simulink model "mg_simulator"  (Simulink 9.0)
settings: Solver=VariableStepAuto  StartTime=0.0  StopTime=Tsim  FixedStep=.005  MaxStep=Ts  RelTol=1e-6  EnableMultiTasking=on
InitFcn:
  | mg_simulator_init
values from neighbouring files (symbols this model uses):
  g_vector = zeros(1,4)    [mg_simulator_init.m]
  Init = [100; 200; 300; 400]    [mg_simulator_init.m]
  N = 2    [mg_simulator_init.m]
  n_Qi = total(2)    [estimator_pflow_dynamics.m]    (also in estimator_pflow_dynamics2.m; mg_simulator_init.m = 4.24e-4*ones(1,4))
  Q = 5*eye    [mg_simulator_init.m]
  Q_di = total(4)    [estimator_pflow_dynamics.m]    (also in estimator_pflow_dynamics2.m; mg_simulator_init.m = 0*ones(1,4))
  Q_Li = 0*ones(1,4)    [mg_simulator_init.m]
  R = 1*eye    [mg_simulator_init.m]
  Thresh = 1    [mg_simulator_init.m]
  Ts = total(7)    [estimator_pflow_dynamics.m]    (also in estimator_pflow_dynamics2.m = total(8); mg_simulator_init.m = 0.005)
  v_ref = 310    [mg_simulator_init.m]
  W = 10*eye    [mg_simulator_init.m]
  w_noise_est = w_noise    [mg_simulator_init.m]
undefined symbols (not defined in the file or in its folder): mpc_run_nodewise_mdl_fast, mpc_run_nodewise_mdl_fast2, mpc_run_nodewise_mdl_fast3, plecs
libraries: sharedTrackingLibrary x4
settings Model: SuppressorTable=22 serialization::archive 11 0 6 0 0 0 0 0  Creator=manaswini  LastModifiedBy=seananderson  ExtModeAutoUpdateStatusClock=off
settings DataIOCC: LimitDataPoints=on  SignalLoggingSaveFormat=ModelDataLogs
settings OptimizationCC: ExpressionDepthLimit=2147483647
settings DebuggingCC: AlgebraicLoopMsg=none  SaveWithParameterizedLinksMsg=none  MaxConsecutiveZCsMsg=none  SolverPrmCheckMsg=warning  FcnCallInpInsideContextMsg=warning  StateNameClashWarn=warning
settings HardwareCC: TargetHWDeviceType=32-bit Generic
settings GRTTargetCC: TargetFcnLib=ansi_tfl_tmw.mat  CombineOutputUpdateFcns=off  GRTInterface=on

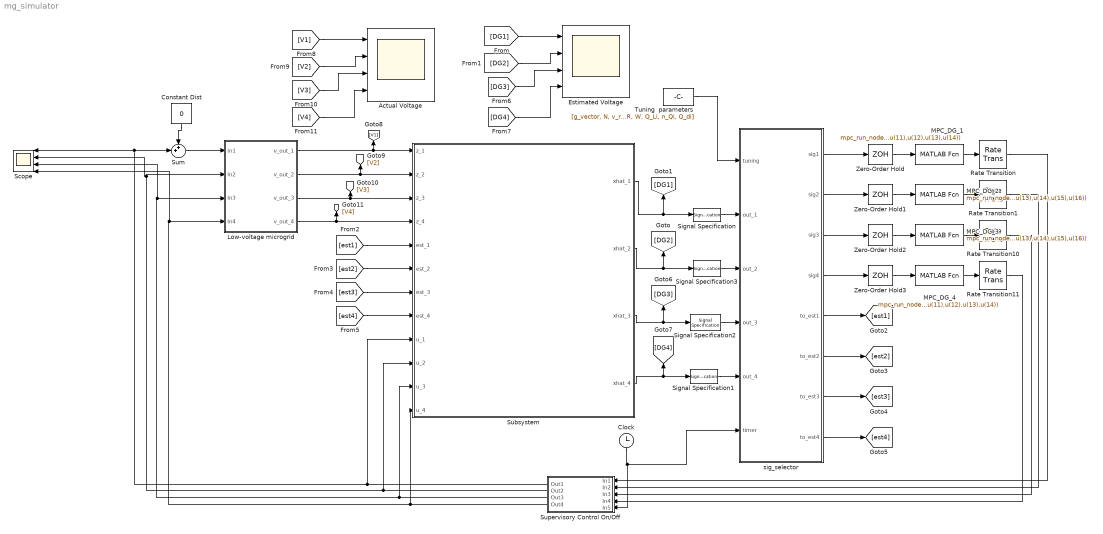
== system mg_simulator ==
  Actual Voltage : Scope  NumInputPorts=4
  Clock : Clock
  Constant Dist : Constant  Value=0
  Estimated Voltage : Scope  NumInputPorts=4
  Low-voltage microgrid : Subsystem  LoadFcn=plecs('sl', 200);  InitFcn=plecs('sl', 214);  StartFcn=plecs('sl', 208);  StopFcn=plecs('sl', 209);  mask(PlecsCircuit){PLECSData=<binary blob, 37876 chars, not shown>}
      mask prompts: PLECSData "PLECS Data (Do not delete or modify!)"
      mask init:
      | % PLACE CUSTOM INITIALIZATIONS ABOVE
      | % DO NOT REMOVE
      | plecs('sl', 215);
      | % DO NOT REMOVE
      settings: CopyFcn=plecs('sl', 203);  DeleteFcn=plecs('sl', 205);  UndoDeleteFcn=plecs('sl', 206);  PreSaveFcn=plecs('sl', 211);  PostSaveFcn=plecs('sl', 201);  NameChangeFcn=plecs('sl', 210);  DestroyFcn=plecs('sl', 207);  PreCopyFcn=plecs('sl', 216);  OpenFcn=plecs('sl', 202);  ErrorFcn=plerrorfcn
      mask Help: web(['file:///' fullfile(plecsdoc, 'creatingacircuit.html')])
      mask Display: disp('PLECS\nCircuit')
  MPC_DG_1 : MATLABFcn  MATLABFcn=mpc_run_nodewise_mdl_fast(u(1),u(2),u(3),u(4),u(5),u(6),u(7),u(8),u(9),u(10),u(11),u(12),u(13),u(14))  SampleTime=Ts
  MPC_DG_2 : MATLABFcn  MATLABFcn=mpc_run_nodewise_mdl_fast2(u(1),u(2:3),u(4:5),u(6),u(7),u(8),u(9),u(10),u(11),u(12),u(13),u(14),u(15),u(16))  SampleTime=Ts
  MPC_DG_3 : MATLABFcn  MATLABFcn=mpc_run_nodewise_mdl_fast3(u(1),u(2:3),u(4:5),u(6),u(7),u(8),u(9),u(10),u(11),u(12),u(13),u(14),u(15),u(16))  SampleTime=Ts
  MPC_DG_4 : MATLABFcn  MATLABFcn=mpc_run_nodewise_mdl_fast(u(1),u(2),u(3),u(4),u(5),u(6),u(7),u(8),u(9),u(10),u(11),u(12),u(13),u(14))  SampleTime=Ts
  Rate Transition{,1,10..11} (4 alike) : RateTransition  OutPortSampleTimeOpt=Inherit  OutPortSampleTime=Ts
  Scope : Scope  NumInputPorts=4
  Signal Specification : SignalSpecification  Dimensions=[ 1 2]
  Signal Specification1 : SignalSpecification  Dimensions=[ 1 2]
  Signal Specification2 : SignalSpecification  Dimensions=[ 1 3]
  Signal Specification3 : SignalSpecification  Dimensions=[ 1 3]
  Subsystem : Subsystem
  Sum : Sum  Inputs=++|
  Supervisory Control On/Off : Subsystem
  Tuning  parameters : Constant  Value=[g_vector, N, v_ref, Ts, Q, R, W, Q_Li, n_Qi, Q_di]
  Zero-Order Hold{,1..3} (4 alike) : ZeroOrderHold  SampleTime=Ts
  sig_selector : MATLAB Function  TreatAsAtomicUnit=on
  wires:
  Clock/1 -> sig_selector/6(timer), Supervisory Control On/Off/5(In5)
  Tuning  parameters/1 -> sig_selector/1(tuning)
  Zero-Order Hold/1 -> MPC_DG_1/1
  sig_selector/1(sig1) -> Zero-Order Hold/1
  MPC_DG_1/1 -> Rate Transition/1
  Rate Transition/1 -> Supervisory Control On/Off/1(In1)
  MPC_DG_2/1 -> Rate Transition1/1
  sig_selector/2(sig2) -> Zero-Order Hold1/1
  Rate Transition1/1 -> Supervisory Control On/Off/2(In2)
  [DG1] -> Estimated Voltage/1
  [DG2] -> Estimated Voltage/2
  sig_selector/5(to_est1) -> [est1]
  sig_selector/6(to_est2) -> [est2]
  Zero-Order Hold1/1 -> MPC_DG_2/1
  Supervisory Control On/Off/1(Out1) -> Subsystem/9(u_1), Sum/2, Scope/1
  Supervisory Control On/Off/2(Out2) -> Subsystem/10(u_2), Low-voltage microgrid/2(In2), Scope/2
  Zero-Order Hold2/1 -> MPC_DG_3/1
  sig_selector/3(sig3) -> Zero-Order Hold2/1
  MPC_DG_3/1 -> Rate Transition10/1
  Zero-Order Hold3/1 -> MPC_DG_4/1
  sig_selector/4(sig4) -> Zero-Order Hold3/1
  MPC_DG_4/1 -> Rate Transition11/1
  sig_selector/7(to_est3) -> [est3]
  sig_selector/8(to_est4) -> [est4]
  Rate Transition10/1 -> Supervisory Control On/Off/3(In3)
  Rate Transition11/1 -> Supervisory Control On/Off/4(In4)
  Supervisory Control On/Off/3(Out3) -> Subsystem/11(u_3), Low-voltage microgrid/3(In3), Scope/3
  Supervisory Control On/Off/4(Out4) -> Subsystem/12(u_4), Low-voltage microgrid/4(In4), Scope/4
  Subsystem/2(xhat_2) -> Signal Specification3/1, [DG2]
  Low-voltage microgrid/1(v_out_1) -> [V1], Subsystem/1(z_1)
  Low-voltage microgrid/3(v_out_3) -> [V3], Subsystem/3(z_3)
  Low-voltage microgrid/4(v_out_4) -> [V4], Subsystem/4(z_4)
  [est1] -> Subsystem/5(est_1)
  [est2] -> Subsystem/6(est_2)
  [est3] -> Subsystem/7(est_3)
  [est4] -> Subsystem/8(est_4)
  Subsystem/4(xhat_4) -> Signal Specification1/1, [DG4]
  Subsystem/3(xhat_3) -> Signal Specification2/1, [DG3]
  [DG3] -> Estimated Voltage/3
  [DG4] -> Estimated Voltage/4
  Signal Specification/1 -> sig_selector/2(out_1)
  Subsystem/1(xhat_1) -> Signal Specification/1, [DG1]
  Signal Specification1/1 -> sig_selector/5(out_4)
  Signal Specification2/1 -> sig_selector/4(out_3)
  Signal Specification3/1 -> sig_selector/3(out_2)
  [V4] -> Actual Voltage/4
  [V3] -> Actual Voltage/3
  [V1] -> Actual Voltage/1
  [V2] -> Actual Voltage/2
  Low-voltage microgrid/2(v_out_2) -> [V2], Subsystem/2(z_2)
  Sum/1 -> Low-voltage microgrid/1(In1)
  Constant Dist/1 -> Sum/1

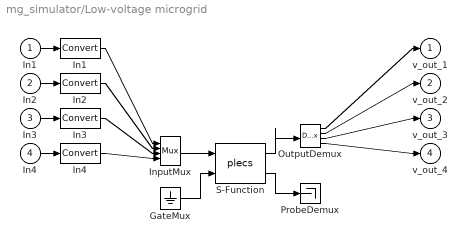
== system mg_simulator/Low-voltage microgrid ==
  In1 : Inport  PortDimensions=1
  In2 : Inport  Port=2  PortDimensions=1
  In3 : Inport  Port=3  PortDimensions=1
  In4 : Inport  Port=4  PortDimensions=1
  " GateMux " : Ground
  " In1 " : DataTypeConversion  SaturateOnIntegerOverflow=on  RndMeth=Zero
  " In2 " : DataTypeConversion  SaturateOnIntegerOverflow=on  RndMeth=Zero
  " In3 " : DataTypeConversion  SaturateOnIntegerOverflow=on  RndMeth=Zero
  " In4 " : DataTypeConversion  SaturateOnIntegerOverflow=on  RndMeth=Zero
  " InputMux " : Mux  Inputs=[ 1 1 1 1 ]
  " OutputDemux " : Demux  Outputs=[ 1 1 1 1 ]
  " ProbeDemux " : Terminator
  " S-Function " : S-Function  FunctionName=plecs  SFunctionDeploymentMode=off  EnableBusSupport=off
  v_out_1 : Outport  PortDimensions=1
  v_out_2 : Outport  Port=2  PortDimensions=1
  v_out_3 : Outport  Port=3  PortDimensions=1
  v_out_4 : Outport  Port=4  PortDimensions=1
  wires:
  " S-Function "/2 -> " ProbeDemux "/1
  " GateMux "/1 -> " S-Function "/2
  " InputMux "/1 -> " S-Function "/1
  " S-Function "/1 -> " OutputDemux "/1
  In1/1 -> " In1 "/1
  " In1 "/1 -> " InputMux "/1
  In2/1 -> " In2 "/1
  " In2 "/1 -> " InputMux "/2
  In3/1 -> " In3 "/1
  " In3 "/1 -> " InputMux "/3
  In4/1 -> " In4 "/1
  " In4 "/1 -> " InputMux "/4
  " OutputDemux "/1 -> v_out_1/1
  " OutputDemux "/2 -> v_out_2/1
  " OutputDemux "/3 -> v_out_3/1
  " OutputDemux "/4 -> v_out_4/1

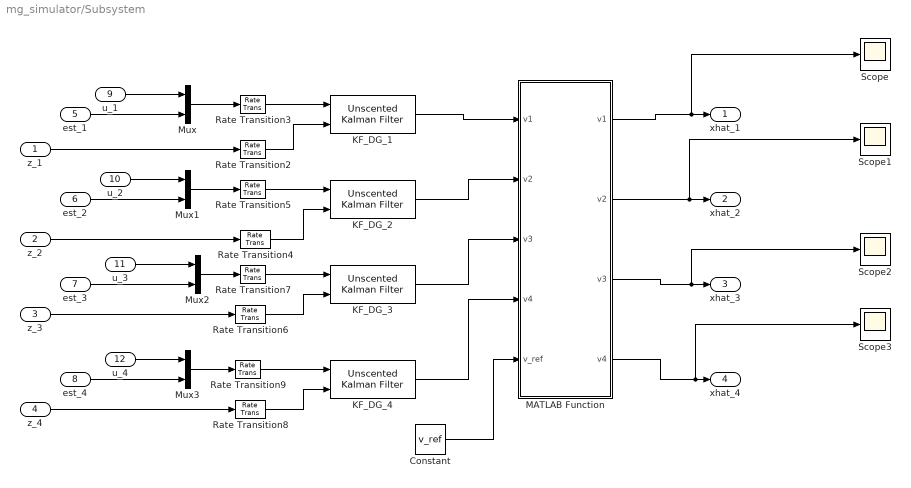
== system mg_simulator/Subsystem ==
  z_1 : Inport
  z_2 : Inport  Port=2
  z_3 : Inport  Port=3
  z_4 : Inport  Port=4
  est_1 : Inport  Port=5
  est_2 : Inport  Port=6
  est_3 : Inport  Port=7
  est_4 : Inport  Port=8
  u_1 : Inport  Port=9
  u_2 : Inport  Port=10
  u_3 : Inport  Port=11
  u_4 : Inport  Port=12
  Constant : Constant  Value=v_ref
  KF_DG_1 : sharedTrackingLibrary/Unscented Kalman Filter  StateTransitionFcn=estimator_pflow_dynamics  HasAdditiveProcessNoise=Nonadditive  ProcessNoise=p_noise_est{i}  HasTimeVaryingProcessNoise=off  HasStateTransitionFcnExtraArgument=1  InitialState=init_state{i}  InitialStateCovariance=p_noise_est{i}  Alpha=1e-1  Beta=2  Kappa=0  MeasurementFcn1=estimator_measurementFcn  HasMeasurementEnablePort1=off  HasAdditiveMeasurementNoise1=Nonadditive  MeasurementNoise1=w_noise_est(i)  HasTimeVaryingMeasurementNoise1=off  HasMeasurementFcnExtraArgument1=0  MeasurementFcn2=myMeasurementFcn  HasMeasurementEnablePort2=off  HasAdditiveMeasurementNoise2=Additive  MeasurementNoise2=1  HasTimeVaryingMeasurementNoise2=off  HasMeasurementFcnExtraArgument2=0  MeasurementFcn3=myMeasurementFcn  HasMeasurementEnablePort3=off  HasAdditiveMeasurementNoise3=Additive  MeasurementNoise3=1  HasTimeVaryingMeasurementNoise3=off  HasMeasurementFcnExtraArgument3=0  MeasurementFcn4=myMeasurementFcn  HasMeasurementEnablePort4=off  HasAdditiveMeasurementNoise4=Additive  MeasurementNoise4=1  HasTimeVaryingMeasurementNoise4=off  HasMeasurementFcnExtraArgument4=0  MeasurementFcn5=myMeasurementFcn  HasMeasurementEnablePort5=off  HasAdditiveMeasurementNoise5=Additive  MeasurementNoise5=1  HasTimeVaryingMeasurementNoise5=off  HasMeasurementFcnExtraArgument5=0  EnableMultirate=off  StateTransitionFcnSampleTime=1  MeasurementFcn1SampleTime=1  MeasurementFcn2SampleTime=1  MeasurementFcn3SampleTime=1  MeasurementFcn4SampleTime=1  MeasurementFcn5SampleTime=1  UseCurrentEstimator=on  OutputStateCovariance=off  DataType=double  SampleTime=Ts  NumberOfMeasurements=1  mask(Unscented Kalman Filter){i=1}
      settings: SourceProductName=Control System Toolbox  SourceProductBaseCode=CT
  KF_DG_2 : sharedTrackingLibrary/Unscented Kalman Filter  StateTransitionFcn=estimator_pflow_dynamics2  HasAdditiveProcessNoise=Nonadditive  ProcessNoise=p_noise_est{i}  HasTimeVaryingProcessNoise=off  HasStateTransitionFcnExtraArgument=1  InitialState=init_state{i}  InitialStateCovariance=p_noise_est{i}  Alpha=1e-1  Beta=2  Kappa=0  MeasurementFcn1=estimator_measurementFcn  HasMeasurementEnablePort1=off  HasAdditiveMeasurementNoise1=Nonadditive  MeasurementNoise1=w_noise_est(i)  HasTimeVaryingMeasurementNoise1=off  HasMeasurementFcnExtraArgument1=0  MeasurementFcn2=myMeasurementFcn  HasMeasurementEnablePort2=off  HasAdditiveMeasurementNoise2=Additive  MeasurementNoise2=1  HasTimeVaryingMeasurementNoise2=off  HasMeasurementFcnExtraArgument2=0  MeasurementFcn3=myMeasurementFcn  HasMeasurementEnablePort3=off  HasAdditiveMeasurementNoise3=Additive  MeasurementNoise3=1  HasTimeVaryingMeasurementNoise3=off  HasMeasurementFcnExtraArgument3=0  MeasurementFcn4=myMeasurementFcn  HasMeasurementEnablePort4=off  HasAdditiveMeasurementNoise4=Additive  MeasurementNoise4=1  HasTimeVaryingMeasurementNoise4=off  HasMeasurementFcnExtraArgument4=0  MeasurementFcn5=myMeasurementFcn  HasMeasurementEnablePort5=off  HasAdditiveMeasurementNoise5=Additive  MeasurementNoise5=1  HasTimeVaryingMeasurementNoise5=off  HasMeasurementFcnExtraArgument5=0  EnableMultirate=off  StateTransitionFcnSampleTime=1  MeasurementFcn1SampleTime=1  MeasurementFcn2SampleTime=1  MeasurementFcn3SampleTime=1  MeasurementFcn4SampleTime=1  MeasurementFcn5SampleTime=1  UseCurrentEstimator=on  OutputStateCovariance=off  DataType=double  SampleTime=Ts  NumberOfMeasurements=1  mask(Unscented Kalman Filter){i=2}
      settings: SourceProductName=Control System Toolbox  SourceProductBaseCode=CT
  KF_DG_3 : sharedTrackingLibrary/Unscented Kalman Filter  StateTransitionFcn=estimator_pflow_dynamics2  HasAdditiveProcessNoise=Nonadditive  ProcessNoise=p_noise_est{i}  HasTimeVaryingProcessNoise=off  HasStateTransitionFcnExtraArgument=1  InitialState=init_state{i}  InitialStateCovariance=p_noise_est{i}  Alpha=1e-1  Beta=2  Kappa=0  MeasurementFcn1=estimator_measurementFcn  HasMeasurementEnablePort1=off  HasAdditiveMeasurementNoise1=Nonadditive  MeasurementNoise1=w_noise_est(i)  HasTimeVaryingMeasurementNoise1=off  HasMeasurementFcnExtraArgument1=0  MeasurementFcn2=myMeasurementFcn  HasMeasurementEnablePort2=off  HasAdditiveMeasurementNoise2=Additive  MeasurementNoise2=1  HasTimeVaryingMeasurementNoise2=off  HasMeasurementFcnExtraArgument2=0  MeasurementFcn3=myMeasurementFcn  HasMeasurementEnablePort3=off  HasAdditiveMeasurementNoise3=Additive  MeasurementNoise3=1  HasTimeVaryingMeasurementNoise3=off  HasMeasurementFcnExtraArgument3=0  MeasurementFcn4=myMeasurementFcn  HasMeasurementEnablePort4=off  HasAdditiveMeasurementNoise4=Additive  MeasurementNoise4=1  HasTimeVaryingMeasurementNoise4=off  HasMeasurementFcnExtraArgument4=0  MeasurementFcn5=myMeasurementFcn  HasMeasurementEnablePort5=off  HasAdditiveMeasurementNoise5=Additive  MeasurementNoise5=1  HasTimeVaryingMeasurementNoise5=off  HasMeasurementFcnExtraArgument5=0  EnableMultirate=off  StateTransitionFcnSampleTime=1  MeasurementFcn1SampleTime=1  MeasurementFcn2SampleTime=1  MeasurementFcn3SampleTime=1  MeasurementFcn4SampleTime=1  MeasurementFcn5SampleTime=1  UseCurrentEstimator=on  OutputStateCovariance=off  DataType=double  SampleTime=Ts  NumberOfMeasurements=1  mask(Unscented Kalman Filter){i=3}
      settings: SourceProductName=Control System Toolbox  SourceProductBaseCode=CT
  KF_DG_4 : sharedTrackingLibrary/Unscented Kalman Filter  StateTransitionFcn=estimator_pflow_dynamics  HasAdditiveProcessNoise=Nonadditive  ProcessNoise=p_noise_est{i}  HasTimeVaryingProcessNoise=off  HasStateTransitionFcnExtraArgument=1  InitialState=init_state{i}  InitialStateCovariance=p_noise_est{i}  Alpha=1e-1  Beta=2  Kappa=0  MeasurementFcn1=estimator_measurementFcn  HasMeasurementEnablePort1=off  HasAdditiveMeasurementNoise1=Nonadditive  MeasurementNoise1=w_noise_est(i)  HasTimeVaryingMeasurementNoise1=off  HasMeasurementFcnExtraArgument1=0  MeasurementFcn2=myMeasurementFcn  HasMeasurementEnablePort2=off  HasAdditiveMeasurementNoise2=Additive  MeasurementNoise2=1  HasTimeVaryingMeasurementNoise2=off  HasMeasurementFcnExtraArgument2=0  MeasurementFcn3=myMeasurementFcn  HasMeasurementEnablePort3=off  HasAdditiveMeasurementNoise3=Additive  MeasurementNoise3=1  HasTimeVaryingMeasurementNoise3=off  HasMeasurementFcnExtraArgument3=0  MeasurementFcn4=myMeasurementFcn  HasMeasurementEnablePort4=off  HasAdditiveMeasurementNoise4=Additive  MeasurementNoise4=1  HasTimeVaryingMeasurementNoise4=off  HasMeasurementFcnExtraArgument4=0  MeasurementFcn5=myMeasurementFcn  HasMeasurementEnablePort5=off  HasAdditiveMeasurementNoise5=Additive  MeasurementNoise5=1  HasTimeVaryingMeasurementNoise5=off  HasMeasurementFcnExtraArgument5=0  EnableMultirate=off  StateTransitionFcnSampleTime=1  MeasurementFcn1SampleTime=1  MeasurementFcn2SampleTime=1  MeasurementFcn3SampleTime=1  MeasurementFcn4SampleTime=1  MeasurementFcn5SampleTime=1  UseCurrentEstimator=on  OutputStateCovariance=off  DataType=double  SampleTime=Ts  NumberOfMeasurements=1  mask(Unscented Kalman Filter){i=4}
      settings: SourceProductName=Control System Toolbox  SourceProductBaseCode=CT
  MATLAB Function : MATLAB Function  TreatAsAtomicUnit=on
  Mux{,1..3} (4 alike) : Mux  Inputs=2
  Rate Transition{2..9} (8 alike) : RateTransition
  Scope{,1..3} (4 alike) : Scope
  xhat_1 : Outport
  xhat_2 : Outport  Port=2
  xhat_3 : Outport  Port=3
  xhat_4 : Outport  Port=4
  wires:
  Rate Transition2/1 -> KF_DG_1/2
  Mux1/1 -> Rate Transition5/1
  est_1/1 -> Mux/2
  z_1/1 -> Rate Transition2/1
  z_2/1 -> Rate Transition4/1
  Rate Transition4/1 -> KF_DG_2/2
  est_2/1 -> Mux1/2
  Mux/1 -> Rate Transition3/1
  u_3/1 -> Mux2/1
  est_4/1 -> Mux3/2
  z_4/1 -> Rate Transition8/1
  z_3/1 -> Rate Transition6/1
  Rate Transition6/1 -> KF_DG_3/2
  Mux2/1 -> Rate Transition7/1
  est_3/1 -> Mux2/2
  Rate Transition8/1 -> KF_DG_4/2
  Mux3/1 -> Rate Transition9/1
  u_4/1 -> Mux3/1
  u_2/1 -> Mux1/1
  u_1/1 -> Mux/1
  Rate Transition3/1 -> KF_DG_1/1
  Rate Transition5/1 -> KF_DG_2/1
  Rate Transition7/1 -> KF_DG_3/1
  Rate Transition9/1 -> KF_DG_4/1
  KF_DG_1/1 -> MATLAB Function/1("v1 ")
  KF_DG_2/1 -> MATLAB Function/2("v2 ")
  KF_DG_3/1 -> MATLAB Function/3("v3 ")
  KF_DG_4/1 -> MATLAB Function/4("v4 ")
  Constant/1 -> MATLAB Function/5(v_ref)
  MATLAB Function/1(v1) -> Scope/1, xhat_1/1
  MATLAB Function/2(v2) -> Scope1/1, xhat_2/1
  MATLAB Function/3(v3) -> Scope2/1, xhat_3/1
  MATLAB Function/4(v4) -> Scope3/1, xhat_4/1

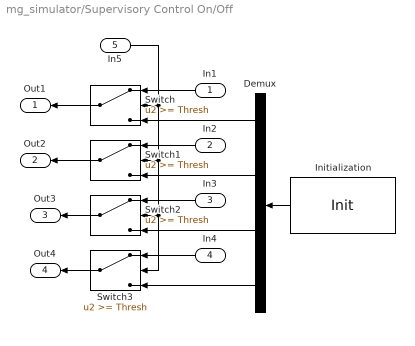
== system mg_simulator/Supervisory Control On/Off ==
  In1 : Inport
  In2 : Inport  Port=2
  In3 : Inport  Port=3
  In4 : Inport  Port=4
  In5 : Inport  Port=5
  Demux : Demux
  Initialization : Constant  Value=Init
  Switch{,1..3} (4 alike) : Switch  Threshold=Thresh
  Out1 : Outport
  Out2 : Outport  Port=2
  Out3 : Outport  Port=3
  Out4 : Outport  Port=4
  wires:
  Demux/2 -> Switch1/3
  Demux/1 -> Switch/3
  Initialization/1 -> Demux/1
  Switch/1 -> Out1/1
  In2/1 -> Switch1/1
  Switch1/1 -> Out2/1
  In5/1 -> Switch3/2, Switch2/2, Switch1/2, Switch/2
  In1/1 -> Switch/1
  Demux/3 -> Switch2/3
  Demux/4 -> Switch3/3
  In3/1 -> Switch2/1
  In4/1 -> Switch3/1
  Switch2/1 -> Out3/1
  Switch3/1 -> Out4/1

== matlab function Subsystem/MATLAB Function ==
  data: v1 input double; v1 output double; v2 input double; v3 input double; v4 input double; v2 output double; v3 output double; v4 output double; v_ref input double
function [v1,v2,v3,v4] = error_update(v1,v2,v3,v4, v_ref)

% update V1
if v1(2) > 1.05*v_ref || v1(2) <= .9*v_ref
    v1(2) = v2(1);
end

%update V2
if any(v2(2:end) > 1.05*v_ref) || any(v2(2:end) <= .9*v_ref)
    v2(2) = v1(1);
    v2(3) = v3(1);
end

%update V3
if any(v3(2:end) > 1.05*v_ref) || any(v3(2:end) <= .9*v_ref)
    v3(2) = v2(1);
    v3(3) = v4(1);
end


% update V4
if v4(2) > 1.05*v_ref || v4(2) <= .9*v_ref
    v4(2) = v3(1);
end

== matlab function sig_selector ==
  data: sig1 output double; tuning input double; out_1 input double; out_2 input double; out_3 input double; out_4 input double; sig2 output double; sig3 output double; sig4 output double; timer input double; to_est1 output double; to_est2 output double; to_est3 output double; to_est4 output double
function [sig1, sig2, sig3, sig4, to_est1, to_est2, to_est3, to_est4] = ...
    selector(tuning, out_1, out_2, out_3, out_4, timer)
% [g_vector, N, v_ref, Ts, Q, R, W, Q_Li, n_Qi, Q_di]
g = tuning(1:4);
N = tuning(5);
v_ref = tuning(6);
Ts = tuning(7);
Q = tuning(8);
R = tuning(9);
W = tuning(10);
Q_L_i = tuning(11:14);
n_Qi = tuning(15:18);
Q_di = tuning(19:22);

% create the signals to send to the distributed MPC algorithms
sig1 = [out_1(1), out_1(2), 2, 1, ...
    N, v_ref(1), n_Qi(1), Q_L_i(1), Q_di(1), Ts, Q, W, R, timer]';
sig2 = [out_2(1), [out_2(2), out_2(3)], [1 3], 2, ...
    N, v_ref, n_Qi(2), Q_L_i(2), Q_di(2), Ts, Q, W, R, timer]';
sig3 = [out_3(1), [out_3(2), out_3(3)], [2 4], 3, ...
    N, v_ref, n_Qi(3), Q_L_i(3), Q_di(3), Ts, Q, W, R, timer]';
sig4 = [out_4(1), out_4(2), 3, 4, ...
    N, v_ref, n_Qi(4), Q_L_i(4), Q_di(4), Ts, Q, W, R, timer]';

% create the signals to send to the estimators
to_est1 = double([n_Qi(1), Q_L_i(1), Q_di(1), 2, 1, Ts]);
to_est2 = double([n_Qi(2), Q_L_i(2), Q_di(2), [1 3], 2, Ts]);
to_est3 = double([n_Qi(3), Q_L_i(3), Q_di(3), [2 4], 3, Ts]);
to_est4 = double([n_Qi(4), Q_L_i(4), Q_di(4), 3, 4, Ts]);
end
